simulink model "massignment7"  (Simulink 6.0)
settings: Solver=FixedStepDiscrete  StartTime=0.0  StopTime=10.0  RelTol=1e-3
libraries: massignmentLib x2
settings Model: Creator=awarlock  LastModifiedBy=awarlock  ExtModeAutoUpdateStatusClock=off
settings OptimizationCC: InlineParams=on
settings DebuggingCC: MultiTaskDSMMsg=warning

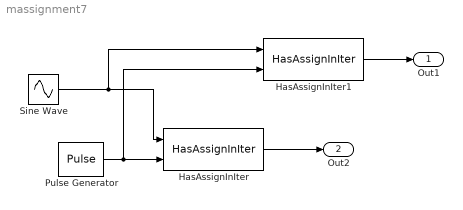
== system massignment7 ==
  HasAssignInIter : massignmentLib/HasAssignInIter
  HasAssignInIter1 : massignmentLib/HasAssignInIter
  Pulse Generator : DiscretePulseGenerator  SampleTime=0.1
  Sine Wave : Sin  Amplitude=3:7  SampleTime=0.1
  Out1 : Outport
  Out2 : Outport  Port=2
  wires:
  Sine Wave/1 -> HasAssignInIter/1, HasAssignInIter1/1
  HasAssignInIter1/1 -> Out1/1
  HasAssignInIter/1 -> Out2/1
  Pulse Generator/1 -> HasAssignInIter/2, HasAssignInIter1/2
